simulink model "ICARO3_orientation_controllo_BIPE"  (R2014a)
settings: Solver=FixedStepDiscrete  SolverMode=MultiTasking  StartTime=0.0  StopTime=inf  FixedStep=0.001  RelTol=1e-3
PreLoadFcn:
  | Icaro_path;
  | 
  | load_param;
  | 
  | %override compute_alloc_inside load_param !!!
  | compute_alloc_esa;
  | 
  | load('mag_calib_sim_HIL.mat');
  | 
  | init_adaptive;
InitFcn:
  | %define fast control loop sample time
  | ST = 0.005;
  | 
  | %define filters
  | s = tf('s');
  | 
  | % Derivator (useful in PID controller)
  | D = 0.01*s/(0.01*s+1);
  | 
  | % LP 2nd order filter
  | LP = 42.88/(3.5*s^2 + 19.6*s + 42.88);
  | 
  | %load new DP position controllers
  | progetto_controllo_pos_v1;
undefined symbols (not defined in the file): DiscIntNeverNeededParam, Earth, G, H, INV_PITCH_RANGE, INV_ROLL_RANGE, INV_THROTTLE_RANGE, INV_YAW_RANGE, PITCH_IDX, PITCH_MID, ROLL_IDX, ROLL_MID, RTOL, THROTTLE_DOWN, THROTTLE_IDX, THROTTLE_LOW_THRES, Ts, WGS84, YAW_IDX, YAW_MID
libraries: simulink x15, GPIO_Lib x3, cstblocks x2, aerolibtransform2 x1, STM32_Config_Lib x1
(part 1 of 5)
settings Model: BufferReuse=off  Creator=reynaudp  LastModifiedBy=ivald
settings DataIOCC: ReturnWorkspaceOutputs=on
settings OptimizationCC: BufferReuse=off  GlobalBufferReuse=off  ExpressionDepthLimit=2147483647  LocalBlockOutputs=off  OptimizeModelRefInitCode=on  LifeSpan=1
settings DebuggingCC: ReadBeforeWriteMsg=DisableAll  WriteAfterWriteMsg=DisableAll  WriteAfterReadMsg=DisableAll  UnderspecifiedInitializationDetection=Classic  MultiTaskDSMMsg=none  FrameProcessingCompatibilityMsg=error  StateNameClashWarn=warning
settings HardwareCC: ProdLargestAtomicInteger=Integer  ProdLargestAtomicFloat=Float  ProdIntDivRoundTo=Zero  ProdEndianess=LittleEndian  ProdHWDeviceType=STMicroelectronics->STM32 32-bit Cortex-M
settings ModelReferenceCC: UpdateModelReferenceTargets=IfOutOfDate
settings SFSimCC: SFSimEcho=off  SimBuildMode=sf_make_clean
settings RTWCC: SystemTargetFile=stm32.tlc  TemplateMakefile=stm32.tmf  Description=stm32 (Embedded Target)  ProcessScript=stm32_make_rtw_hook  CodeProfilingSaveOptions=AllData  CheckMdlBeforeBuild=Warning
settings RTWCC: CustomSource=|
  | stm32f4xx_hal_can.c
  | stm32f4xx_hal_tim.c
  | stm32f4xx_hal_tim_ex.c
  | stm32f4xx_hal_i2c.c
  | stm32f4xx_hal_uart.c
  | stm32f4xx_hal_adc.c
  | stm32f4xx_hal_adc_ex.c
  | 
  | circular_buffer.c
  | stm32f4_custom_USART.c
  | stm32f4_I2C1_sensors.c
  | stm32f4_I2C1_peripheral.c
  | stm32f4_LED_debug.c
  | 
  | packet_manager.c
  | packet_manager_c2k_car.c
  | packet_command.c
  | packet_command_tel.c
  | packet_gps.c
  | 
  | packet_telemetry.c
  | packet_status.c
  | packet_telemetry_LF.c
  | packet_debug_6_floats.c
  | packet_telemetry_type.c
  | packet_statistics_telemetry.c
  | packet_statistics_i2c_telemetry.c
  | packet_attitude.c
  | packet_waypoint.c
  | packet_fuzzyguidance.c
  | 
  | packet_bs_telemetry.c packet_car_telemetry.c
  | packet_pc_to_bs.c packet_bs_to_car.c
  | 
  | packet_gps_time.c
  | packet_startstop_seeker.c
  | packet_startstop_seeker_init.c
  | packet_pc_to_car.c
settings CodeAppCC: IgnoreCustomStorageClasses=off  MaxIdLength=64  CustomSymbolStrType=$N$R$M  MATLABSourceComments=on  InternalIdentifier=Classic
settings STFCustomTargetCC: ParMdlRefBuildCompliant=on  ConcurrentExecutionCompliant=off  IncludeMdlTerminateFcn=off  GeneratePreprocessorConditionals=Use local settings  CombineOutputUpdateFcns=on  ERTCustomFileBanners=on  SupportContinuousTime=off  SupportNonInlinedSFcns=off  SupportVariableSizeSignals=on  MATLABClassNameForMDSCustomization=Simulink.SoftwareTarget.ERTCustomization  GRTInterface=off  SystemTargetFile=stm32.tlc
settings ERTTargetCC: GenerateSampleERTMain=off  ParMdlRefBuildCompliant=on  IncludeMdlTerminateFcn=off  SupportVariableSizeSignals=on  InlinedParameterPlacement=Hierarchical  ERTSrcFileBannerTemplate=sourceFileTemplate.cgt  ERTHdrFileBannerTemplate=sourceFileTemplate.cgt  ERTDataSrcFileTemplate=sourceFileTemplate.cgt  ERTDataHdrFileTemplate=sourceFileTemplate.cgt  ERTCustomFileTemplate=customRoutineProcess_RTOS.tlc

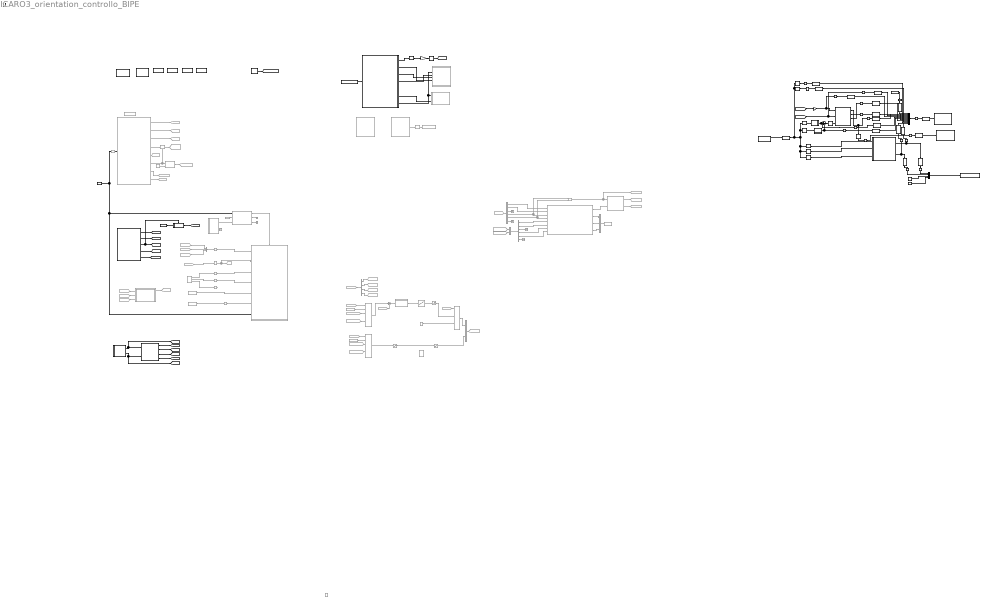
== system ICARO3_orientation_controllo_BIPE ==
  note: yaw
  note: clock
      | RPY
      | Gyro
      | Accelerometro
      | Tag0
      | Tag1
      | ACC
      | GYRO
      | robotpose
      | waypoint
      | steer
      | throttle
  note: // 0: lat
      |                         // 1: lon
      |                         // 2: status
      |                         // 3: speed over ground
      |                         // 4: course over ground
      |                         // 5: gps quality indicator
      |                         // 6: number of satellites
      |                         // 7: hdop
      |                         // 8: altitude
      |                         // 9: dgps station id
  note: GPS
  note: Wireless com
      | (not in use)
  note: ADNS 3080
  note: PC for live inspection
      | OpenLog to log data
  note: from v.5: Porting by PepiPa
  note: ICARO III Firmware
  note: RIDEFINIZIONE HANDLER INTERRUZIONI
      | Commentare gli handler definiti nel file
      | <install_dir>\STM32F4xx-MAT\STM32F4xx\src\stm32f4xx_it.c
      |
      | Fatto per:
      | - I2C1_EV_IRQHandler()
      | - I2C1_ER_IRQHandler()
  note: CONFIGURAZIONE GPS
      | Baud Rate: 115200
      | USART 6
      | PIN: PC6->TX    PC7->RX
      | Message type: UBX
      |
      | Assicurarsi che sia configurato
      | così
  note: CONFIGURAZIONE MAGNETOMETRO
      | I2C1
      | SDA: PB9
      | SCL: PB6
  note: Modalità di funzionamento indicate dalla variabile "mode":
      | 0:  mototi fermi => PWM = 0 per sterzo e trazione
      | 1: Guida LOS, senza PI, solo sullo sterzo, il segnale PWM per la trazione è inviato da pc
      | 2: PI con alta saturazione sull'integrale (anti-windup)
      | 3: PI con saturazione moderata (utilizzata in seguito per il firmaware definitivo)
      | 4: motori comandati direttamente da pc, sia sterzo che trazione
      | defult: motori fermi.
      |
      | Se non viene ricevuto alcun pacchetto per 1 secondo i PWM vanno a 0
  note: TX Diagram: Agent to Base Station
  note: RX Diagram: Base Station to Agent
  note: 1 - SENSORs DATA ACQUISITION
  note: GUIDANCE SYSTEM (PNG)
  note: BMS: Battery Manegament Unit (ADC)
  note: Hardware Settings
  note: CONFIGURAZIONE GPS
      | Baud Rate: 9600
      | Message type: binary
      |
      | Assicurarsi che sia configurato
      | così
  note: USART3: PC
      | RX: PC11
      | TX: PC10
      | Baud: 115200
  note: DEBUG SENSORI
      | Aggiungere nel codice
      | #define I2C1_SENSORS_TEST
  note: I2C1
      | SDA: PB9
      | SCL: PB6
  note: PWM-LED
      | Pin 12, 13, 14, 15
  note: USART2: XBEE
      | RX: PA3
      | TX: PA2
      | Baud: 57600
  note: USART4:  Arduino
      | RX: PA1
      | TX: PA0
      | Baud: 57600
  note: USART5: GPS
      | RX: PD2
      | TX: PC12
      | Baud: 115200
  note: 2 - NAVIGATION SYSTEM
  note: 3 - KINEMATICS: CAR POSITION CONTROLLER
  note: 4.1 - DYNAMICS: THROTTLE SPEED CONTROLLER (PID/OL)
  note: ( HOMING GUIDANCE )
  note: ( OPEN-LOOP, POINT TO POINT, TRACKING )
  note: valori costanti che vanno bene:
      | Vy=0.1 e Vx=--0.2 oppure il contrario
      | oppure Vy=-0.2 Vx=0.4
      | il vincolo è che il modulo sia piccolo
      | sennò deve crescere la v del seeker
      | che però è già al limite. Per quanto riguarda gamma
      | iniziale, la situazione migliore è che il seeker parta sulla stessa y del target
      | e orientato verso di lui. Al limite variare l orientazione di poco come nell' ini
      | _2. Invece nel ini_3 le y dei due veicoli non coincidono ma differiscono
      | di 5 metri ed in più il seeker non parte orientato verso il target. Fondamentale:
      | puoi assumere anche velocità target di quasi 1 m/s in modulo, ma è importante
      | che il seeker non parta orientato in modo che, ad un certo punto, si possa trovare
      | parallelo al target. ATTENZIONE QUINDI A 2 FATTORI:
      | 1-target non troppo veloce
      | 2-seeker orientato all' inizio abbastanza verso il target
  note: Modalità di funzionamento indicate dalla variabile "mode":
      | 0: Stop
      | 1: Guidance
      | 2:
      | 3: Waypoint
      | 4:Openloop
  note: 4.2 - DYNAMICS: STEER POSITION CONTROLLER (OL)
  note: il limite di 0.25 è dovuto
      | al limite di sterzata ammissibile
      | dalla brontosaurus, ovvero circa
      | pi/12.
  note: [-0.2 0 0.2] rad
      | [700,1500,2300]us - eps
      |
      | eps = 10us, due to zero crossing
  note: if error > 1 m/s,
      | Go to maximum velociy..
      |
      | FIX WITH A GOOD LOOKUP TABLE
  note: Fix the velocity to V/2
      | if the objective is Follow a Track
      | ( Its not properly tracking )
  note: Send to telemetry
  note: Data coming from Intel Joule:
      | - 1:3 -> (x,y,z) tag0
      | - 4:6 -> (x,y,z) tag1
      | - 7:9 -> (x,y,z) waypoint
      | - 10 -> startstop
      | - 11:13 -> (x,y,theta) robot_pose
  note: GUIDA WAYPOINT PER VEICOLI SU RUOTE
  " generatore di riferimenti" : Subsystem  Commented=on
  1: HW 0: SIM : Constant
  ADC1 : Subsystem
  ADIS AHRS2 : Subsystem
  Compensate for sensor mount _acc : MATLAB Function  TreatAsAtomicUnit=on
  Compensate for sensor mount _acc1 : MATLAB Function  TreatAsAtomicUnit=on
  Constant ( SIMULATION ONLY ) : Constant  Value=[0 10 50 100 150 200]
  Constant1 : Constant  Commented=on  Value=[0 0]
  Constant2 : Constant  Commented=on  Value=0
  Constant32 : Constant  Value=0
  Constant33 : Constant  Value=0
  "Control " : Subsystem
  DEBUG_DOWNLINK1 : S-Function  Commented=on  FunctionName=sfun_raw_float_downlink  Parameters=0.01  EnableBusSupport=off
  Data Type Conversion mx2 : DataTypeConversion  Commented=on  OutDataTypeStr=single  RndMeth=Round  SaturateOnIntegerOverflow=on
  Data Type Conversion mx3 : DataTypeConversion  OutDataTypeStr=double  RndMeth=Round  SaturateOnIntegerOverflow=on
  Data Type Conversion{1..2,4..7,18,20,22,24..27} (13 alike) : DataTypeConversion  OutDataTypeStr=single  SaturateOnIntegerOverflow=on
  Data Type Conversion16 : DataTypeConversion  OutDataTypeStr=double
  Data Type Conversion17 : DataTypeConversion  OutDataTypeStr=single
  Data Type Conversion19 : DataTypeConversion  OutDataTypeStr=double
  Data Type Conversion3 : DataTypeConversion  OutDataTypeStr=single
  Demux : Demux  Commented=on  Outputs=6
  Demux1 : Demux  Commented=on  Outputs=6
  Demux2 : Demux  Commented=on
  Digital Clock : DigitalClock  SampleTime=0.01
  Digital Clock1 : DigitalClock
  From : From  Commented=on  GotoTag=gps_pos_vel
  From1 : From  Commented=on  GotoTag=v_throttle_ref_png  TagVisibility=global
  From10 : From  Commented=on  GotoTag=GPS_clock  TagVisibility=global
  From14 : From  Commented=on  GotoTag=ref_pos_ecef  TagVisibility=global
  From15 : From  Commented=on  GotoTag=ACC_ADXL  TagVisibility=global
  From16 : From  Commented=on  GotoTag=ref_velocity  TagVisibility=global
  From17 : From  Commented=on  GotoTag=GYRO_ITG  TagVisibility=global
  From18 : From  Commented=on  GotoTag=MAG_HMC  TagVisibility=global
  From2 : From  Commented=on  GotoTag=MAG_HMC  TagVisibility=global
  From3 : From  Commented=on  GotoTag=GPS_data_ECEF  TagVisibility=global
  From4 : From  Commented=on  GotoTag=v_ned_nav  TagVisibility=global
  From5 : From  Commented=on  GotoTag=mode  TagVisibility=global
  From6 : From  Commented=on  GotoTag=gain_pid  TagVisibility=global
  From7 : From  Commented=on  GotoTag=mode  TagVisibility=global
  From8 : From  Commented=on  GotoTag=mode  TagVisibility=global
  From9 : From  Commented=on  GotoTag=GPS_flag  TagVisibility=global
  GET PPS : Subsystem  Commented=on
  GPS receiver : Subsystem
  Gain1 : Gain  Gain=2
  Gain2 : Gain  Gain=1/10
  Goto10 : Goto  Commented=on  GotoTag=gain_pid  TagVisibility=global
  Goto11 : Goto  Commented=on  GotoTag=ref_velocity  TagVisibility=global
  Goto12 : Goto  Commented=on  GotoTag=mode  TagVisibility=global
  Goto14 : Goto  Commented=on  GotoTag=ref_position_ECEF  TagVisibility=global
  Goto16 : Goto  Commented=on  GotoTag=packet_received_flag  TagVisibility=global
  Goto17 : Goto  Commented=on  GotoTag=pwm_pc_openloop  TagVisibility=global
  Goto18 : Goto  Commented=on  GotoTag=pwm_closedloop  TagVisibility=global
  Goto20 : Goto  Commented=on  GotoTag=v_throttle_ref_png  TagVisibility=global
  Goto21 : Goto  Commented=on  GotoTag=v_ned_nav  TagVisibility=global
  Goto22 : Goto  Commented=on  GotoTag=theta_steer_ref_png  TagVisibility=global
  Goto24 : Goto  Commented=on  GotoTag=Kp_throttle  TagVisibility=global
  Goto26 : Goto  Commented=on  GotoTag=Ki_throttle  TagVisibility=global
  Goto27 : Goto  Commented=on  GotoTag=RPY_SS  TagVisibility=global
  Goto29 : Goto  Commented=on  GotoTag=Kp_steer  TagVisibility=global
  Goto30 : Goto  Commented=on  GotoTag=Ki_steer  TagVisibility=global
  Goto7 : Goto  Commented=on  GotoTag=mag_xyz  TagVisibility=global
  Goto8 : Goto  Commented=on  GotoTag=ref_pos_ecef  TagVisibility=global
  Goto9 : Goto  Commented=on  GotoTag=waypoint_ned  TagVisibility=global
  "ID CAR " : Constant  SampleTime=-1
  Math Function : Math  Commented=on  Operator=hypot  SaturateOnIntegerOverflow=on
  Multiport Switch2 : MultiPortSwitch  Commented=on  DataPortOrder=Zero-based contiguous  Inputs=5
  Multiport Switch3 : MultiPortSwitch  Commented=on  DataPortOrder=Zero-based contiguous  Inputs=5
  Multiport Switch4 : MultiPortSwitch  Commented=on  DataPortOrder=Zero-based contiguous  Inputs=5
  Mux2 : Mux  Commented=on  Inputs=3
  Mux22 : Mux
  Mux23 : Mux  Inputs=[1 3 3 3 3 3 3 3 3 3 1 1]
  Mux3 : Mux  Commented=on  Inputs=2
  Mux4 : Mux  Commented=on  Inputs=2
  Mux5 : Mux  Commented=on  Inputs=3
  PI Controller : Subsystem  Commented=on
  "Posca_Zocco Steer Map " : Subsystem  Commented=on
  Prescaler : Subsystem  Commented=on
  Pulse Generator : DiscretePulseGenerator  Commented=on  PulseType=Time based  Amplitude=400  Period=20  PulseWidth=50
  Rate Transition{,2,5,8..9,11} (6 alike) : RateTransition  Commented=on
  Rate Transition{1,3..4,6..7,12,44,46..48,50..56} (17 alike) : RateTransition
  Rate Transition10 : RateTransition  Commented=through
  Rate Transition49 : RateTransition  OutPortSampleTime=0.005
  S-Function-USART3_Receive4 : S-Function  FunctionName=sfun_UPboard  EnableBusSupport=off
  S-Function1 : S-Function  Commented=on  FunctionName=sfun_pm_init_car  EnableBusSupport=off
  S-Function2 : S-Function  Commented=on  FunctionName=sfun_recv_from_bs  EnableBusSupport=off
  SS AHRS : Subsystem  Commented=on
  STM32_Config : STM32_Config_Lib/STM32_Config  Priority=0  Project_Path=C:\Users\ivald\Desktop\BIPE MATLAB\IOC\  Config_File=ICAROIII.ioc  MCU_Name=STM32F407VGTx
  Save data to data logger (the micro SD card)1 : S-Function  FunctionName=sfun_UPboard_downlink  EnableBusSupport=off
  Save data to data logger (the micro SD card)2 : S-Function  FunctionName=sfun_raw_float_downlink  Parameters=0.1  EnableBusSupport=off
  Scheme Running : Subsystem
  Selector1 : Selector  InputPortWidth=3  Indices=[3:3]
  Selector15 : Selector  InputPortWidth=13  Indices=[4:6]
  Selector16 : Selector  InputPortWidth=13  Indices=[7:9]
  Selector2 : Selector  InputPortWidth=13  Indices=[11:13]
  Selector3 : Selector  IndexMode=Zero-based  InputPortWidth=12  Indices=[0:3]
  Selector4 : Selector  InputPortWidth=13  Indices=[10]
  Selector5 : Selector  InputPortWidth=13  Indices=[11:13]
  Selector6 : Selector  InputPortWidth=13  Indices=[7:9]
  Selector8 : Selector  InputPortWidth=13  Indices=[1:3]
  Sum : Sum  Commented=on  Inputs=|+-
  Sum12 : Sum  Inputs=|+-
  Terminator{,1..6} (7 alike) : Terminator  Commented=on
  Theta_Sat @ 0.25 rad : Saturate  Commented=on  UpperLimit=0.25  LowerLimit=-0.25
  To Workspace2 : ToWorkspace  Commented=on  VariableName=ENG  SaveFormat=Structure With Time  SampleTime=-1
  USART2 Initialization : S-Function  FunctionName=sfun_USART2_Init  EnableBusSupport=off
  USART3 Initialization : S-Function  FunctionName=sfun_USART3_Init  EnableBusSupport=off
  USART4 Initialization : S-Function  FunctionName=sfun_USART4_Init  EnableBusSupport=off
  USART5 Initialization : S-Function  FunctionName=sfun_USART5_Init  EnableBusSupport=off
  V/2 : Constant  Commented=on  Value=1600
  "[V0,VMAX] Saturation" : Saturate  Commented=on  UpperLimit=1750  LowerLimit=1450
  "[rad]" : From  Commented=on  GotoTag=theta_steer_ref_png  TagVisibility=global
  "[rad]1" : From  Commented=on  GotoTag=v_throttle_ref_waypoint
  "[rad]2" : From  Commented=on  GotoTag=theta_steer_ref_waypoint
  blocco motori se non arrivano pacchetti : Subsystem  Commented=on
  clock latch : Subsystem  TreatAsAtomicUnit=on
  configurazione relativa seeker/target : Subsystem  Commented=on
  debug telemtry FLIGHT TEST : Subsystem  Commented=on
  debug telemtry FLIGHT TEST1 : Subsystem  Commented=on
  debug telemtry STATIC TEST : Subsystem  Commented=on
  debug_telemetry_minimal : Subsystem  Commented=on
  latch1 : Subsystem  Commented=on  TreatAsAtomicUnit=on
  m/s 2 usec : Lookup_n-D  Commented=on  NumberOfTableDimensions=1  BreakpointsForDimension1=[0 1]  Table=[1450 1750]  RndMeth=Simplest  InputSameDT=on
  offset : Constant  Commented=on  Value=0
  power computations1 : Subsystem
  pwm & pi cmds : Subsystem  Commented=on
  "rad 2 usec Lookup Table " : Lookup  Commented=on  InputValues=[-1.57, 0, 1.57]  Table=[690,1490,2290]  SaturateOnIntegerOverflow=on
  reproduce PWM9 : S-Function  FunctionName=sfun_PWM_servomotor  Parameters=ST,1,1,1,1  EnableBusSupport=off
  second to stop : Constant  Commented=on
  send gps to bs : Subsystem  Commented=on
  sensor and actuators interface : Subsystem
  v_0 : Constant  Commented=on  Value=0
  v_1 : Constant  Commented=on  Value=0
  Constant : Constant  IOType=siggen
  tag scope: GPS_3dfix_age=global, GPS_age=global, GPS_clock=global, GPS_data=global, GPS_data_ECEF=global, GPS_flag=global, HW_SIM_selector=global, I_batt=global, I_batt_filt=global, I_consumption_Ah=global, P_batt_filt=global, V_batt=global, V_batt_filt=global, radio_ch=global
  wires:
  Gain2/1 -> Selector3/1
  sensor and actuators interface/3(Error Counter) -> debug telemtry FLIGHT TEST/4(JETI error counter)
  Selector3/1 -> [radio_ch]
  Data Type Conversion mx3/1 -> Gain2/1
  sensor and actuators interface/4(i2c debug) -> debug telemtry FLIGHT TEST/3(i2c debug)
  GPS receiver/2(GPS age) -> [GPS_age]
  sensor and actuators interface/6(i2c errors management) -> debug telemtry STATIC TEST/2(i2c errors)
  GPS receiver/1(GPS data) -> [GPS_data]
  sensor and actuators interface/1(pwms [us]) -> Data Type Conversion mx3/1
  sensor and actuators interface/2(rc age) -> debug telemtry FLIGHT TEST/5(Rc age)
  sensor and actuators interface/7(i2c enable flags) -> debug telemtry STATIC TEST/1(i2c enable flags), debug telemtry FLIGHT TEST/2(i2c enable flags)
  GPS receiver/4(GPS 3D fix age) -> [GPS_3dfix_age]
  Data Type Conversion mx2/1 -> DEBUG_DOWNLINK1/1
  SS AHRS/1(RPY_SS) -> Goto27/1
  From15/1 -> SS AHRS/1(ACC)
  From17/1 -> SS AHRS/2(PQR)
  From18/1 -> SS AHRS/3(MAG)
  ADC1/1(V_batt) -> [V_batt], power computations1/1(V)
  ADC1/2(I_batt) -> [I_batt], power computations1/2(I)
  power computations1/1(V_filt) -> [V_batt_filt]
  power computations1/2(I_filt) -> [I_batt_filt]
  power computations1/3(P_ist) -> [P_batt_filt]
  power computations1/4(I_integ) -> [I_consumption_Ah]
  debug_telemetry_minimal/1(to telemetry TX) -> Data Type Conversion mx2/1
  Constant ( SIMULATION ONLY )/1 -> sensor and actuators interface/1(motors_cmd)
  GET PPS/1(PPS pulse) -> Prescaler/3(PPS PULSE)
  offset/1 -> Prescaler/2(offset [ms])
  Prescaler/2(counter value before reset) -> Terminator1/1
  GET PPS/2(PPS TIME ublox) -> Terminator/1
  Prescaler/3(counter value) -> Terminator2/1
  From2/1 -> Rate Transition2/1
  Rate Transition5/1 -> send gps to bs/1(GPS to send)  "0: ecef_px  1: ecef_py: 2: ecef_pz  3: ecef_vx 4: ecef_vy 5: ecef_vz  6: gps_fiix 7:fix_time"
  Rate Transition2/1 -> send gps to bs/2(MAG to send), Goto7/1  "0: mag_x 1: mag_y 2: mag_z"
  pwm & pi cmds/1(mode) -> Rate Transition/1
  pwm & pi cmds/2(pi_cmds) -> Rate Transition8/1
  pwm & pi cmds/3(pwm) -> Rate Transition9/1
  Constant2/1 -> Rate Transition11/1
  Rate Transition/1 -> send gps to bs/3(execution mode)  "Mode € [0,5]"
  Rate Transition8/1 -> send gps to bs/4(pid_command)  "[Kp, Ki]"
  Rate Transition9/1 -> ?
  Rate Transition11/1 -> send gps to bs/6(heading_error)  "Heading_Error"
  Rate Transition10/1 -> S-Function2/1  "ID"
  "ID CAR "/1 -> Rate Transition10/1, send gps to bs/7(id_car), Prescaler/1(ID time slot)  "ID"
  From3/1 -> Mux2/1  "( x, x_dot )"
  From9/1 -> Mux2/2  "Flag"
  Mux2/1 -> Rate Transition5/1
  GPS receiver/3(GPS data valid flag) -> clock latch/Enable, [GPS_flag]
  Digital Clock/1 -> clock latch/1(In)
  clock latch/1(Out) -> [GPS_clock]
  From10/1 -> Mux2/3  "Ck"
  second to stop/1 -> blocco motori se non arrivano pacchetti/2(second to stop)
  S-Function2/1 -> Goto12/1  "Mode € [0,5] FROM BS"
  S-Function2/2 -> Goto8/1
  S-Function2/6 -> blocco motori se non arrivano pacchetti/1(pck arrived), latch1/Enable
  S-Function2/4 -> latch1/1(In1)  "PWM DIrect Command"
  S-Function2/5 -> Goto10/1
  S-Function2/3 -> Goto9/1
  S-Function2/8 -> Goto11/1
  S-Function2/7 -> Goto14/1
  1: HW 0: SIM/1 -> [HW_SIM_selector]
  Constant1/1 -> send gps to bs/5(pwm command)
  blocco motori se non arrivano pacchetti/1(stop) -> Goto16/1
  latch1/1(Out1) -> Goto17/1
  configurazione relativa seeker/target/4(Rdot) -> Mux5/3
  configurazione relativa seeker/target/3(sigma dot) -> Mux5/2
  Demux1/6 -> Terminator6/1
  Demux1/5 -> configurazione relativa seeker/target/8(vy_t_ECEF)
  Demux1/4 -> configurazione relativa seeker/target/7(vx_t_ECEF)
  Mux3/1 -> Demux1/1
  From16/1 -> Mux3/2
  Demux1/3 -> Terminator5/1
  From14/1 -> Mux3/1
  Demux/4 -> Math Function/1, configurazione relativa seeker/target/3(vx_s_ECEF)
  Mux5/1 -> To Workspace2/1
  Demux/6 -> Terminator4/1
  configurazione relativa seeker/target/1(a_c) -> " generatore di riferimenti"/2(a_c)
  Demux/2 -> configurazione relativa seeker/target/2(y_s_ECEF)
  Demux/3 -> Terminator3/1
  Demux/1 -> configurazione relativa seeker/target/1("x_s_ECEF ")
  configurazione relativa seeker/target/2(R) -> Mux5/1
  Demux1/1 -> configurazione relativa seeker/target/5(x_t_ECEF)
  Demux1/2 -> configurazione relativa seeker/target/6(y_t_ECEF)
  Demux/5 -> Math Function/2, configurazione relativa seeker/target/4(vy_s_ECEF)
  From/1 -> Demux/1
  Math Function/1 -> Goto21/1, " generatore di riferimenti"/1(V_istantanea)
  " generatore di riferimenti"/1(V_ref) -> Goto20/1
  " generatore di riferimenti"/2(sterzo_ref) -> Goto22/1
  Mux4/1 -> Goto18/1
  m/s 2 usec/1 -> "[V0,VMAX] Saturation"/1
  From4/1 -> Sum/2
  "rad 2 usec Lookup Table "/1 -> Mux4/2
  Theta_Sat @ 0.25 rad/1 -> "rad 2 usec Lookup Table "/1
  Multiport Switch3/1 -> Theta_Sat @ 0.25 rad/1
  From5/1 -> Multiport Switch2/1
  v_0/1 -> Multiport Switch2/2
  From1/1 -> Multiport Switch2/3
  "[rad]1"/1 -> Multiport Switch2/5
  From8/1 -> Multiport Switch3/1
  v_1/1 -> Multiport Switch3/2
  "[rad]"/1 -> Multiport Switch3/3
  "[rad]2"/1 -> Multiport Switch3/5
  Multiport Switch2/1 -> Sum/1  "v_ref"
  Sum/1 -> PI Controller/1(Vref-Vk)  "e"
  PI Controller/1(V_out= K*e) -> m/s 2 usec/1  "k*e"
  From7/1 -> Multiport Switch4/1
  "[V0,VMAX] Saturation"/1 -> Multiport Switch4/3
  V/2/1 -> Multiport Switch4/5
  Multiport Switch4/1 -> Mux4/1
  From6/1 -> Demux2/1
  Demux2/3 -> Goto29/1
  Demux2/4 -> Goto30/1
  Demux2/1 -> Goto24/1
  Demux2/2 -> Goto26/1
  Prescaler/1(START TO SEND) -> send gps to bs/Enable  "CK"
  GPS receiver/5(GPS data ECEF) -> [GPS_data_ECEF]
  Data Type Conversion18/1 -> Selector6/1, Selector2/1, Selector15/1, Selector8/1, Selector4/1, Selector16/1, Selector5/1
  Selector8/1 -> Compensate for sensor mount _acc/1(u)  "tag0"
  Selector15/1 -> Compensate for sensor mount _acc1/1(u)  "tag1"
  S-Function-USART3_Receive4/1 -> Data Type Conversion18/1
  Selector16/1 -> "Control "/2(waypoint)  "(x,y) waypoint"
  Selector5/1 -> "Control "/1("robotpose ")  "robotpose"
  Selector4/1 -> "Control "/3(startstop)  "startstop"
  Rate Transition49/1 -> ADIS AHRS2/3(MAG)
  Sum12/1 -> Rate Transition49/1  "heading direction"
  Constant33/1 -> Mux22/3
  Constant32/1 -> Mux22/4
  Rate Transition46/1 -> Rate Transition3/1
  Data Type Conversion16/1 -> Rate Transition48/1
  Data Type Conversion19/1 -> Rate Transition47/1
  Rate Transition47/1 -> Mux22/1
  [GYRO_MPU] -> ADIS AHRS2/2(PQR), Rate Transition53/1
  Rate Transition44/1 -> Data Type Conversion17/1
  Mux22/1 -> reproduce PWM9/1
  Data Type Conversion17/1 -> Save data to data logger (the micro SD card)2/1
  Mux23/1 -> Rate Transition44/1
  Rate Transition50/1 -> Data Type Conversion22/1
  Rate Transition55/1 -> Data Type Conversion24/1
  Rate Transition56/1 -> Data Type Conversion25/1
  ADIS AHRS2/1(RPY_ADIS) -> Rate Transition54/1, Selector1/1  "yaw"
  Rate Transition51/1 -> Data Type Conversion20/1
  ADIS AHRS2/3(debiased PQR) -> Rate Transition55/1
  ADIS AHRS2/2(ACC_NED) -> Rate Transition56/1
  Rate Transition52/1 -> Data Type Conversion26/1
  [ACC_MPU] -> Gain1/1
  Rate Transition53/1 -> Data Type Conversion27/1
  Compensate for sensor mount _acc/1(y) -> Rate Transition51/1, Sum12/1
  Compensate for sensor mount _acc1/1(y) -> Rate Transition50/1, Sum12/2
  Gain1/1 -> Rate Transition52/1, ADIS AHRS2/1(ACC)
  Digital Clock1/1 -> Rate Transition1/1
  Rate Transition54/1 -> Data Type Conversion1/1
  Data Type Conversion27/1 -> Mux23/3
  Data Type Conversion26/1 -> Mux23/4
  Data Type Conversion20/1 -> Mux23/5
  Data Type Conversion22/1 -> Mux23/6
  Data Type Conversion25/1 -> Mux23/7
  Data Type Conversion24/1 -> Mux23/8
  Rate Transition1/1 -> Data Type Conversion2/1
  Data Type Conversion1/1 -> Mux23/2
  Data Type Conversion2/1 -> Mux23/1
  "Control "/1("steer ") -> Rate Transition12/1, Data Type Conversion19/1
  "Control "/2(throttle) -> Rate Transition7/1, Data Type Conversion16/1
  Selector1/1 -> Rate Transition46/1
  Rate Transition3/1 -> Data Type Conversion3/1
  Data Type Conversion3/1 -> Save data to data logger (the micro SD card)1/1
  Selector2/1 -> Rate Transition4/1
  Data Type Conversion4/1 -> Mux23/9
  Rate Transition4/1 -> Data Type Conversion4/1
  Selector6/1 -> Rate Transition6/1
  Rate Transition6/1 -> Data Type Conversion5/1
  Data Type Conversion5/1 -> Mux23/10
  Rate Transition48/1 -> Mux22/2
  Data Type Conversion6/1 -> Mux23/11
  Data Type Conversion7/1 -> Mux23/12
  Rate Transition7/1 -> Data Type Conversion7/1
  Rate Transition12/1 -> Data Type Conversion6/1

== system ICARO3_orientation_controllo_BIPE/ generatore di riferimenti ==
  V_istantanea : Inport
  a_c : Inport  Port=2
  fcn : MATLAB Function  TreatAsAtomicUnit=on
  V_ref : Outport
  sterzo_ref : Outport  Port=2
  wires:
  fcn/2(sterzo_ref) -> sterzo_ref/1
  V_istantanea/1 -> fcn/1(V_istantanea)
  a_c/1 -> fcn/2(a_c)
  fcn/1(V_ref) -> V_ref/1

== system ICARO3_orientation_controllo_BIPE/ADC1 ==
  Current sensor sensitivity : Constant  Commented=on  Value=0.028 * 3.3 / 5
  Data Type Conversion : DataTypeConversion
  Data Type Conversion1 : DataTypeConversion  Commented=on  OutDataTypeStr=single  SaturateOnIntegerOverflow=on
  Data Type Conversion3 : DataTypeConversion  Commented=on  OutDataTypeStr=single  SaturateOnIntegerOverflow=on
  Demux : Demux
  Gain1 : Gain  Commented=on  Gain=3/4096
  Gain16 : Gain  Commented=on  Gain=3/4096
  Gain2 : Gain  Commented=on  Gain=3/4096
  Mux : Mux  Commented=on
  PWM1 : S-Function  FunctionName=sfun_ADC_Receive  Parameters=0.01  EnableBusSupport=off
  PWM2 : S-Function  Commented=on  FunctionName=sfun_show_ADC  EnableBusSupport=off
  Product : Product  Commented=on  Inputs=*/  RndMeth=Zero
  Rate Transition : RateTransition  OutPortSampleTime=0.01
  S-Function1 : S-Function  Commented=on  FunctionName=sfun_raw_float_downlink  Parameters=0.01  EnableBusSupport=off
  S-Function4 : S-Function  Commented=on  FunctionName=sfun_raw_float_downlink  Parameters=0.01  EnableBusSupport=off
  Sum : Sum  Commented=on  Inputs=|+-
  scale factor for resistor network - from direct V measures : Gain  Commented=on  Gain=16.43/1.69
  scale factor for resistor network - from mesarured R1 and R2 : Gain  Gain=(9.06 + 1.122)/1.122  SampleTime=0.01
  V_batt : Outport
  I_batt : Outport  Port=2
  tag scope: ADC_A0=global, ADC_A1=global, ADC_A2=global, ADC_A3=global
  wires:
  Gain16/1 -> scale factor for resistor network - from direct V measures/1
  Demux/2 -> Gain1/1, Mux/2, [ADC_A1]
  Demux/3 -> Gain2/1, Mux/3, [ADC_A2]
  scale factor for resistor network - from direct V measures/1 -> V_batt/1
  Gain1/1 -> Sum/1  "V_meas"
  Gain2/1 -> Sum/2  "V_ref"
  Sum/1 -> Product/1
  Current sensor sensitivity/1 -> Product/2
  Product/1 -> I_batt/1
  Demux/4 -> Mux/4, [ADC_A3]
  PWM1/1 -> PWM2/1, Data Type Conversion/1
  Data Type Conversion/1 -> Rate Transition/1
  Demux/1 -> Mux/1, [ADC_A0], Gain16/1
  Data Type Conversion3/1 -> S-Function4/1
  Mux/1 -> Data Type Conversion3/1
  Data Type Conversion1/1 -> S-Function1/1
  Rate Transition/1 -> Data Type Conversion1/1, Demux/1

== system ICARO3_orientation_controllo_BIPE/ADIS AHRS2 ==
  ACC : Inport
  PQR : Inport  Port=2
  MAG : Inport  Port=3
  Attitude Filter ADIS : Subsystem  mask{T=ST}
      mask prompts: T "Sample Time"
  Constant1 : Constant  Value=[0 0 0]'  OutDataTypeStr=Inherit: Inherit via back propagation
  Data Type Conversion mx1 : DataTypeConversion  OutDataTypeStr=single  RndMeth=Round  SaturateOnIntegerOverflow=on
  Data Type Conversion mx10 : DataTypeConversion  OutDataTypeStr=double  RndMeth=Round  SaturateOnIntegerOverflow=on
  Data Type Conversion mx17 : DataTypeConversion  OutDataTypeStr=double  RndMeth=Round  SaturateOnIntegerOverflow=on
  Data Type Conversion mx2 : DataTypeConversion  OutDataTypeStr=single  RndMeth=Round  SaturateOnIntegerOverflow=on
  Data Type Conversion mx3 : DataTypeConversion  OutDataTypeStr=single  RndMeth=Round  SaturateOnIntegerOverflow=on
  Terminator : Terminator
  Terminator1 : Terminator
  debias ADIS : Subsystem
  debias ADIS1 : Subsystem  Commented=on
  RPY_ADIS : Outport
  ACC_NED : Outport  Port=2
  debiased PQR : Outport  Port=3
  filter running : Outport  Port=4
  wires:
  Attitude Filter ADIS/1(q) -> Terminator1/1
  Attitude Filter ADIS/3(gyro_bias) -> Terminator/1
  Data Type Conversion mx17/1 -> debiased PQR/1
  Data Type Conversion mx10/1 -> RPY_ADIS/1
  Attitude Filter ADIS/4(a_ned) -> ACC_NED/1
  ACC/1 -> debias ADIS/1(acc)
  debias ADIS/3(detrending_ok) -> Attitude Filter ADIS/Enable, filter running/1
  debias ADIS/2(gyro_out) -> Data Type Conversion mx2/1
  debias ADIS/1(acc_out) -> Data Type Conversion mx1/1
  MAG/1 -> Data Type Conversion mx3/1
  Attitude Filter ADIS/2(rpy) -> Data Type Conversion mx10/1
  Constant1/1 -> Attitude Filter ADIS/4(bias)
  PQR/1 -> debias ADIS/2(gyros)
  Data Type Conversion mx1/1 -> Attitude Filter ADIS/1(acc)
  Data Type Conversion mx2/1 -> Attitude Filter ADIS/3(gyro), Data Type Conversion mx17/1
  Data Type Conversion mx3/1 -> Attitude Filter ADIS/2(mag)

== system ICARO3_orientation_controllo_BIPE/Control  ==
  "robotpose " : Inport
  waypoint : Inport  Port=2
  startstop : Inport  Port=3
  " (x,y)" : Selector  Indices=[1:2]
  (x,y) : Selector  Indices=[1:2]
  Data Type Conversion1 : DataTypeConversion  OutDataTypeStr=double
  Data Type Conversion2 : DataTypeConversion  OutDataTypeStr=double
  Data Type Conversion3 : DataTypeConversion  OutDataTypeStr=double
  Data Type Conversion4 : DataTypeConversion  OutDataTypeStr=single
  Data Type Conversion5 : DataTypeConversion  OutDataTypeStr=single
  Gain : Gain  Gain=1000
  Sum2 : Sum  Inputs=|+-
  Sum3 : Sum  Inputs=-+|
  VectorNorm : MATLAB Function  TreatAsAtomicUnit=on
  atan2 : MATLAB Function  TreatAsAtomicUnit=on
  steer_control : Subsystem
  "throttle_control " : Subsystem
  yaw_amcl : Selector  Indices=[3]
  "steer " : Outport
  throttle : Outport  Port=2
  wires:
  (x,y)/1 -> atan2/1(u)  "angle_error"
  Sum2/1 -> (x,y)/1, " (x,y)"/1  "relative vector"
  VectorNorm/1(y) -> steer_control/1(distance_to_waypoint), "throttle_control "/1(distance_to_waypoint)  "distance to waypoint"
  " (x,y)"/1 -> Gain/1  "(x,y)"
  waypoint/1 -> Data Type Conversion2/1
  "robotpose "/1 -> Data Type Conversion1/1
  startstop/1 -> Data Type Conversion3/1
  Data Type Conversion3/1 -> steer_control/3(startstop), "throttle_control "/2(startstop)
  Data Type Conversion5/1 -> "steer "/1
  "throttle_control "/1(thrrottle) -> Data Type Conversion4/1
  Data Type Conversion4/1 -> throttle/1
  steer_control/1("steer ") -> Data Type Conversion5/1
  Data Type Conversion2/1 -> Sum2/1
  Data Type Conversion1/1 -> yaw_amcl/1, Sum2/2
  Gain/1 -> VectorNorm/1(u)
  atan2/1(theta) -> Sum3/2
  Sum3/1 -> steer_control/2(rel_angle)
  yaw_amcl/1 -> Sum3/1

== system ICARO3_orientation_controllo_BIPE/GET PPS ==
  Data Type Conversion6 : DataTypeConversion  OutDataTypeStr=uint16  LockScale=on
  Demux : Demux  Outputs=16
  Digital Clock : DigitalClock  SampleTime=-1
  GPIO_Read : GPIO_Lib/GPIO_Read  Port_name=GPIOD  Pin_0=on  Pin_1=off  Pin_2=off  Pin_3=off  Pin_4=off  Pin_5=off  Pin_6=off  Pin_7=off  Pin_8=off  Pin_9=off  Pin_10=off  Pin_11=off  Pin_12=off  Pin_13=off  Pin_14=off  Pin_15=off  PinList=GPIOD0
  GPIO_Write : GPIO_Lib/GPIO_Write  Port_name=GPIOD  Pin0=off  Toggle_Pin0=off  Pin1=off  Toggle_Pin1=off  Pin2=off  Toggle_Pin2=off  Pin3=off  Toggle_Pin3=off  Pin4=off  Toggle_Pin4=off  Pin5=off  Toggle_Pin5=off  Pin6=off  Toggle_Pin6=off  Pin7=off  Toggle_Pin7=off  Pin8=off  Toggle_Pin8=off  Pin9=off  Toggle_Pin9=off  Pin10=off  Toggle_Pin10=off  Pin11=off  Toggle_Pin11=off  Pin12=off  Toggle_Pin12=off  Pin13=off  Toggle_Pin13=off  Pin14=on  Toggle_Pin14=off  Pin15=off  Toggle_Pin15=off  PinList="GPIOD12  13  14  15"
  Signal Specification : SignalSpecification
  clock latch : Subsystem  TreatAsAtomicUnit=on
  step 2 pulse : Subsystem
  uint16 to vector : MATLAB Function  TreatAsAtomicUnit=on
  PPS pulse : Outport
  PPS TIME ublox : Outport  Port=2
  wires:
  Signal Specification/1 -> uint16 to vector/1(gpioD)
  Digital Clock/1 -> clock latch/1(In)
  Demux/1 -> step 2 pulse/1(step)
  step 2 pulse/1(pulse) -> PPS pulse/1, clock latch/Enable
  clock latch/1(Out) -> PPS TIME ublox/1
  uint16 to vector/1(out) -> Demux/1
  GPIO_Read/1 -> GPIO_Write/1, Data Type Conversion6/1  "Toggle PD14 if PPS ARRIVEs"
  Data Type Conversion6/1 -> Signal Specification/1

== system ICARO3_orientation_controllo_BIPE/GPS receiver ==
  note: GPS_data (index zero-based):
      | 0: latitude
      | 1: longitude:
      | 2: fix_mode
      | 8: altitude
  note: gps_data_valid
      | signal values are:
      | 0: no packet received
      | 1: packet received
  note: // 0: lat
      |                         // 1: lon
      |                         // 2: status
      |                         // 3: speed over ground
      |                         // 4: course over ground
      |                         // 5: gps quality indicator
      |                         // 6: number of satellites
      |                         // 7: hdop
      |                         // 8: altitude
      |                         // 9: dgps station id
  note: NOTE: GPS age measure the age of a packet
      | regardless of the fact that the packet contains valid data
      | (that is a fix_quality not 0) or not
      | Thus it can be used ONLY for detection of gps presence
      | or malfunctioning (no packets sent) during flight
      | and NOT for determining the availability of a good gps fix
  note: GPS DATA 16 STANDARD FORMAT
      | 0: lat
      | 1: lon
      | 2: status  {0: nofix, 1:2D, 2:3D, 3:3D+SBAS }
      | 3: speed over ground
      | 4: course over ground
      | 5: gps quality indicator
      | 6: number of satellites
      | 7: hdop
      | 8: altitude
      | 9: dgps station id
      | 10: ECEF Position x
      | 11: ECEF Position y
      | 12: ECEF Position z
      | 13: ECEF Velocity x
      | 14: ECEF Velocity y
      | 15: ECEF Velocity z
  Demux : Demux  Outputs=[10 6]
  Product : Product  RndMeth=Zero
  UBLOX LEA 6 GPS : Subsystem
  VENUS GPS : Subsystem  Commented=on
  compute 3d age : Subsystem
  compute age : Subsystem
  get fix_quality_flag : Selector  IndexMode=Zero-based  InputPortWidth=10  Indices=2
  gps selector 1 : ManualSwitch  CurrentSetting=0
  gps selector 2 : ManualSwitch  CurrentSetting=0
  GPS data : Outport
  GPS age : Outport  Port=2
  GPS data valid flag : Outport  Port=3
  GPS 3D fix age : Outport  Port=4
  GPS data ECEF : Outport  Port=5
  wires:
  compute age/1(gps_arrived_flag_out) -> GPS data valid flag/1
  compute age/2(gps_arrived_age) -> GPS age/1
  compute 3d age/1(gps_3d_fix_age) -> GPS 3D fix age/1
  Product/1 -> compute 3d age/1(gps_fix_quality_flag)
  get fix_quality_flag/1 -> Product/2
  VENUS GPS/2(sync_pulse) -> gps selector 2/1
  VENUS GPS/1(gps_data_16) -> gps selector 1/1
  gps selector 2/1 -> compute age/1(gps_arrived_flag), Product/1
  gps selector 1/1 -> Demux/1
  UBLOX LEA 6 GPS/1(GPS data_16) -> gps selector 1/2
  UBLOX LEA 6 GPS/2(sync_pulse) -> gps selector 2/2
  Demux/1 -> get fix_quality_flag/1, GPS data/1
  Demux/2 -> GPS data ECEF/1

== system ICARO3_orientation_controllo_BIPE/PI Controller ==
  Vref-Vk : Inport
  Compare To Constant : simulink/Logic and Bit Operations/Compare To Constant  relop===  const=3  OutDataTypeStr=boolean
  Discrete-Time Integrator : DiscreteIntegrator  ExternalReset=rising  SampleTime=-1  LimitOutput=on  UpperSaturationLimit=1  LowerSaturationLimit=0  ICPrevOutput=DiscIntNeverNeededParam  ICPrevScaledInput=DiscIntNeverNeededParam
  Product : Product
  Product1 : Product
  Sum1 : Sum  Inputs=|++
  V_out= K*e : Outport
  wires:
  Sum1/1 -> V_out= K*e/1
  Product1/1 -> Sum1/1
  [Ki_throttle] -> Product/1
  Vref-Vk/1 -> Product/2, Product1/1
  [mode] -> Compare To Constant/1
  Product/1 -> Discrete-Time Integrator/1
  Discrete-Time Integrator/1 -> Sum1/2
  Compare To Constant/1 -> Discrete-Time Integrator/2
  [Kp_throttle] -> Product1/2

== system ICARO3_orientation_controllo_BIPE/Posca_Zocco Steer Map  ==
  note: la x è la coordinata trasversale,
      | la y quella longitudinale per andare avnti o indietro.
      |
      | la y è presa così come è, soltanto limitata tra 1 e -1;
      |
      | la x invece è moltiplicata per -0.182 così i valori in uscita sono
      | limitati tra 0.2 e -0.2
      | in quanto i valori che entrano da 'In1' sono al più uguali
      | a +1 o -1.
  Command2PWM : Gain  Commented=on  Gain=-273/1500
  From5 : From  Commented=on  GotoTag=theta_steer_ref
  Normalization @[-1,1] : Lookup  Commented=on  InputValues=[-0.25,0,0.25]  Table=[-1, 0, 1]  SaturateOnIntegerOverflow=on
  Sat @ 0.25 rad : Saturate  Commented=on  UpperLimit=0.25  LowerLimit=-0.25
  Saturation1 : Saturate  Commented=on  UpperLimit=1750  LowerLimit=1220
  mappa sterzo : Lookup  Commented=on  InputValues=[-0.2,0,0.2]  Table=[1220,1485,1750]  SaturateOnIntegerOverflow=on
  Out1 : Outport
  wires:
  Saturation1/1 -> Out1/1
  mappa sterzo/1 -> Saturation1/1
  Normalization @[-1,1]/1 -> Command2PWM/1
  Sat @ 0.25 rad/1 -> Normalization @[-1,1]/1
  Command2PWM/1 -> mappa sterzo/1
  From5/1 -> Sat @ 0.25 rad/1

== system ICARO3_orientation_controllo_BIPE/Prescaler ==
  note: Ipotesi: il periodo con cui parlano gli agenti + basestation
      | è di 200 ms, si considerano 9 macchine + 1 basestation,
      | quindi in totale ogni slot temporale dura 20 ms.
      | Questo schema permette di trovare quando è il momento di inviare i dati.
  note: In ingresso ho un impulso della durata
      | di un colpo di clock, ossia di 1ms.
      |
      | L'integratore non fa altro che sommare 1 ogni millisecondo.
      | Quando arriva l'impulso l'integratore si resetta a 0.
      | Quindi l'integratore conterebbe, se il PPS fosse esattamente
      | di 1 secondo, fino a 999, per poi tornare a 0.
      |
      | Il sottosistema "find send time", trova, in base all'ID
      | della macchina e ad un evenutale offset, quando arriva il
      | momento in cui inviare i dati
  ID time slot : Inport
  offset [ms] : Inport  Port=2
  PPS PULSE : Inport  Port=3
  Unit Delay : UnitDelay  SampleTime=-1
  contatore con reset : DiscreteIntegrator  gainval=1/0.001  ExternalReset=rising  InitialConditionSource=external  SampleTime=-1  ICPrevOutput=DiscIntNeverNeededParam  ICPrevScaledInput=DiscIntNeverNeededParam
  find send time : Subsystem
  latch : Subsystem  TreatAsAtomicUnit=on
  reset value : Constant  Value=0  SampleTime=-1
  to sum : Constant  SampleTime=-1
  START TO SEND : Outport
  counter value before reset : Outport  Port=2
  counter value : Outport  Port=3
  wires:
  to sum/1 -> contatore con reset/1
  reset value/1 -> contatore con reset/3
  PPS PULSE/1 -> contatore con reset/2, latch/Enable
  contatore con reset/1 -> find send time/1("pulse time [ms] "), counter value/1, Unit Delay/1
  latch/1(Out1) -> counter value before reset/1
  Unit Delay/1 -> latch/1(In1)
  ID time slot/1 -> find send time/2(ID car)
  offset [ms]/1 -> find send time/3(Offset [ms])
  find send time/1(start to send) -> START TO SEND/1

== system ICARO3_orientation_controllo_BIPE/SS AHRS ==
  ACC : Inport
  PQR : Inport  Port=2
  MAG : Inport  Port=3
  Attitude Filter SS : Subsystem  mask{T=ST}
      mask prompts: T "Sample Time"
  Constant1 : Constant  Value=[0 0 0]'  OutDataTypeStr=single
  Data Type Conversion mx1 : DataTypeConversion  OutDataTypeStr=single  RndMeth=Round  SaturateOnIntegerOverflow=on
  Data Type Conversion mx10 : DataTypeConversion  OutDataTypeStr=double  RndMeth=Round  SaturateOnIntegerOverflow=on
  Data Type Conversion mx17 : DataTypeConversion  OutDataTypeStr=double  RndMeth=Round  SaturateOnIntegerOverflow=on
  Data Type Conversion mx2 : DataTypeConversion  OutDataTypeStr=single  RndMeth=Round  SaturateOnIntegerOverflow=on
  Data Type Conversion mx4 : DataTypeConversion  OutDataTypeStr=single  RndMeth=Round  SaturateOnIntegerOverflow=on
  Terminator : Terminator
  Terminator1 : Terminator
  debias SS : Subsystem
  RPY_SS : Outport
  ACC_NED : Outport  Port=2
  debiased PQR : Outport  Port=3
  filter running : Outport  Port=4
  wires:
  Constant1/1 -> Attitude Filter SS/4(bias)
  Attitude Filter SS/2(rpy) -> Data Type Conversion mx10/1
  Data Type Conversion mx4/1 -> Attitude Filter SS/2(mag)
  Data Type Conversion mx1/1 -> Attitude Filter SS/1(acc)
  Data Type Conversion mx2/1 -> Data Type Conversion mx17/1, Attitude Filter SS/3(gyro)
  debias SS/3(detrending_ok) -> filter running/1, Attitude Filter SS/Enable
  PQR/1 -> debias SS/2(gyros)
  ACC/1 -> debias SS/1(acc)
  Attitude Filter SS/4(a_ned) -> ACC_NED/1
  Data Type Conversion mx10/1 -> RPY_SS/1
  Data Type Conversion mx17/1 -> debiased PQR/1
  Attitude Filter SS/3(gyro_bias) -> Terminator/1
  Attitude Filter SS/1(q) -> Terminator1/1
  MAG/1 -> Data Type Conversion mx4/1
  debias SS/1(acc_out) -> Data Type Conversion mx1/1
  debias SS/2(gyro_out) -> Data Type Conversion mx2/1

== system ICARO3_orientation_controllo_BIPE/Scheme Running ==
  note: Led toggling = Simulink scheme running in STM32
  GPIO_Write : GPIO_Lib/GPIO_Write  Port_name=GPIOD  Pin0=off  Toggle_Pin0=off  Pin1=off  Toggle_Pin1=off  Pin2=off  Toggle_Pin2=off  Pin3=off  Toggle_Pin3=off  Pin4=off  Toggle_Pin4=off  Pin5=off  Toggle_Pin5=off  Pin6=off  Toggle_Pin6=off  Pin7=off  Toggle_Pin7=off  Pin8=off  Toggle_Pin8=off  Pin9=off  Toggle_Pin9=off  Pin10=off  Toggle_Pin10=off  Pin11=off  Toggle_Pin11=off  Pin12=on  Toggle_Pin12=off  Pin13=off  Toggle_Pin13=off  Pin14=off  Toggle_Pin14=off  Pin15=off  Toggle_Pin15=off  PinList="GPIOD12  13  14  15"
  Pulse Generator1 : DiscretePulseGenerator  PulseType=Time based  Period=0.05  PulseWidth=60
  wires:
  Pulse Generator1/1 -> GPIO_Write/1

== system ICARO3_orientation_controllo_BIPE/blocco motori se non arrivano pacchetti ==
  pck arrived : Inport
  second to stop : Inport  Port=2
  Digital Clock : DigitalClock  SampleTime=-1
  Enabled Subsystem : Subsystem  TreatAsAtomicUnit=on
  Relational Operator : RelationalOperator  Operator=<=  OutDataTypeStr=boolean
  Sum : Sum  Inputs=|-+
  stop : Outport
  wires:
  Digital Clock/1 -> Sum/2, Enabled Subsystem/1(In1)
  Enabled Subsystem/1(Out1) -> Sum/1
  pck arrived/1 -> Enabled Subsystem/Enable
  Sum/1 -> Relational Operator/1
  Relational Operator/1 -> stop/1
  second to stop/1 -> Relational Operator/2

== system ICARO3_orientation_controllo_BIPE/clock latch ==
  In : Inport
  Enable : EnablePort
  Out : Outport  InitialOutput=-1000
  wires:
  In/1 -> Out/1

== system ICARO3_orientation_controllo_BIPE/configurazione relativa seeker//target ==
  "x_s_ECEF " : Inport
  y_s_ECEF : Inport  Port=2
  vx_s_ECEF : Inport  Port=3
  vy_s_ECEF : Inport  Port=4
  x_t_ECEF : Inport  Port=5
  y_t_ECEF : Inport  Port=6
  vx_t_ECEF : Inport  Port=7
  vy_t_ECEF : Inport  Port=8
  engagement : Subsystem
  engagement 2 : Subsystem
  "pure PNG " : Subsystem
  a_c : Outport
  R : Outport  Port=2
  sigma dot : Outport  Port=3
  Rdot : Outport  Port=4
  wires:
  "x_s_ECEF "/1 -> engagement/1(x_s_ECEF)
  y_s_ECEF/1 -> engagement/2(y_s_ECEF)
  vx_s_ECEF/1 -> engagement/5(vx_s_ECEF)
  x_t_ECEF/1 -> engagement/3("x_t_ECEF ")
  y_t_ECEF/1 -> engagement/4(y_t_ECEF)
  vy_s_ECEF/1 -> engagement/6(vy_s_ECEF)
  engagement/1(R) -> R/1
  engagement/3(sigma dot) -> sigma dot/1, "pure PNG "/2("sigma dot ")
  engagement/2(Rdot) -> engagement 2/1(Rdot), Rdot/1
  engagement 2/1(Closing Velocity) -> "pure PNG "/1(Closing velocity)
  "pure PNG "/1(a_c) -> a_c/1
  vx_t_ECEF/1 -> engagement/7(vx_t_ECEF)
  vy_t_ECEF/1 -> engagement/8("vy_t_ECEF ")
